simulink model "model_car"  (R2013b)
settings: Solver=ode45  StartTime=0.0  StopTime=2  FixedStep=0.001  RelTol=1e-3
libraries: cstblocks x6
settings Model: Creator=daniel  LastModifiedBy=daniel
settings ModelReferenceCC: ModelReferenceNumInstancesAllowed=Single

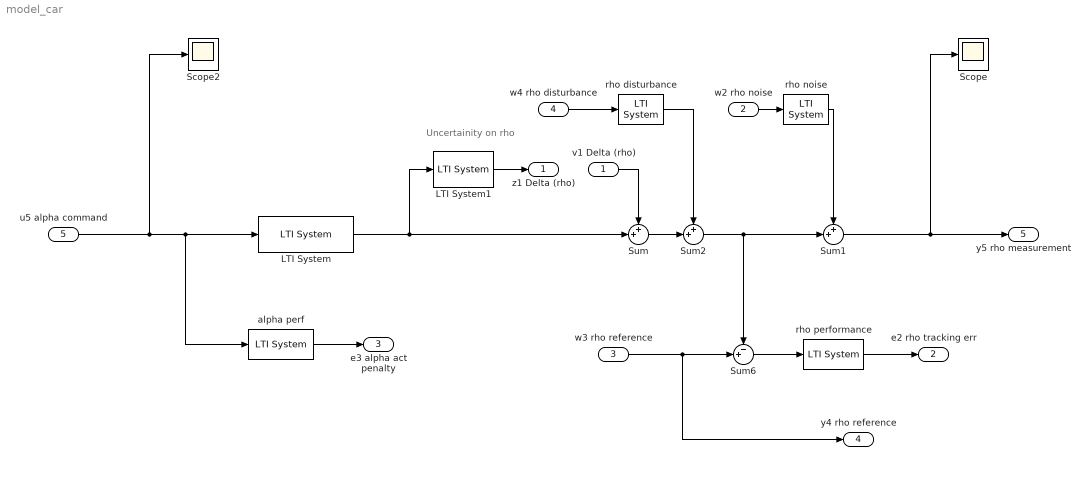
== system model_car ==
  note: Uncertainity on rho
  v1 Delta (rho) : Inport
  w2 rho noise : Inport  Port=2
  w3 rho reference : Inport  Port=3
  w4 rho disturbance : Inport  Port=4
  u5 alpha command : Inport  Port=5
  LTI System : cstblocks/LTI System  sys=P_car  IC=[]
  LTI System1 : cstblocks/LTI System  sys=W_rho  IC=[]
  Scope : Scope
  Scope2 : Scope
      settings: SaveName=ScopeData8
  Sum : Sum  Inputs=++|
  Sum1 : Sum  Inputs=++|
  Sum2 : Sum  Inputs=++|
  Sum6 : Sum  Inputs=-+|
  alpha perf : cstblocks/LTI System  sys=W_alphaperf  IC=[]
  rho disturbance : cstblocks/LTI System  sys=W_rhod  IC=[]
  rho noise : cstblocks/LTI System  sys=W_rhon  IC=[]
  rho performance : cstblocks/LTI System  sys=W_rhoperf  IC=[]
  z1 Delta (rho) : Outport
  e2 rho tracking err : Outport  Port=2
  e3 alpha act penalty : Outport  Port=3
  y4 rho reference : Outport  Port=4
  y5 rho measurement : Outport  Port=5
  wires:
  LTI System/1 -> LTI System1/1, Sum/2
  LTI System1/1 -> z1 Delta (rho)/1
  v1 Delta (rho)/1 -> Sum/1
  u5 alpha command/1 -> Scope2/1, alpha perf/1, LTI System/1
  w2 rho noise/1 -> rho noise/1
  rho noise/1 -> Sum1/1
  Sum1/1 -> Scope/1, y5 rho measurement/1
  w4 rho disturbance/1 -> rho disturbance/1
  rho disturbance/1 -> Sum2/1
  Sum/1 -> Sum2/2
  Sum2/1 -> Sum6/1, Sum1/2
  w3 rho reference/1 -> Sum6/2, y4 rho reference/1
  Sum6/1 -> rho performance/1
  rho performance/1 -> e2 rho tracking err/1
  alpha perf/1 -> e3 alpha act penalty/1
